simulink model "TP3_simulink"  (R2024a)
settings: Solver=VariableStepAuto  StartTime=0.0  StopTime=10  MaxStep=0.001  RelTol=1e-3
values from neighbouring files (symbols this model uses):
  A = [-1/(4*10^-3) -0.1/(4*10^-3) 0; 0.1/(2*10^-3) -(3*10^-3)/(2*10^-3) 0; 0 1 0]    [TP1.m]    (also in TP2.m = [0 1 0 0 0 0; -Kx/m -dx/m 0 0 0 0; 0 0 0 1 0 0; 0 0 -Ky/m -d; TP3.m = [0 1 0 0 0 0; -Kx/m -dx/m 0 0 0 0; 0 0 0 1 0 0; 0 0 -Ky/m -d)
  B = [1/(4*10^-3);0;0]    [TP1.m]    (also in TP2.m = [0 0 0; 1/m 0 0; 0 0 0; 0 1/m 0; 0 0 0; 0 0 1/m]; TP3.m = [0 0 0; 1/m 0 0; 0 0 0; 0 1/m 0; 0 0 0; 0 0 1/m])
  C = [0 0 1]    [TP1.m]    (also in TP2.m = [1 0 0 0 0 0; 0 0 1 0 0 0; 0 0 0 0 1 0]; TP3.m = [1 0 0 0 0 0; 0 0 1 0 0 0; 0 0 0 0 1 0])
  KxC = place(A(1:2,1:2),B(1:2,1),pcmdX)    [TP3.m]
  KyC = place(A(3:4,3:4),B(3:4,2),pcmdY)    [TP3.m]
  KzC = place(A(5:6,5:6),B(5:6,3),pcmdZ)    [TP3.m]
  L = [832330; 691770; 1550]    [TP1.m]    (also in TP2.m = (place(Aob.', C.', p)).'; TP3.m = (place(A.', C.', p)).')
settings Model: Creator=pedro.campos-afonso-  LastModifiedBy=pedro.campos-afonso-

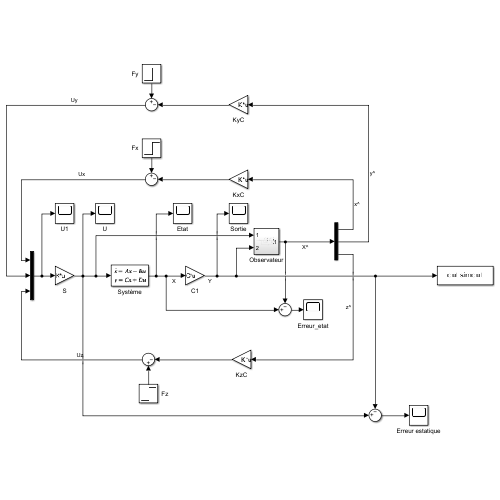
[thumbnail: Simulink's stored preview of the top-level diagram]
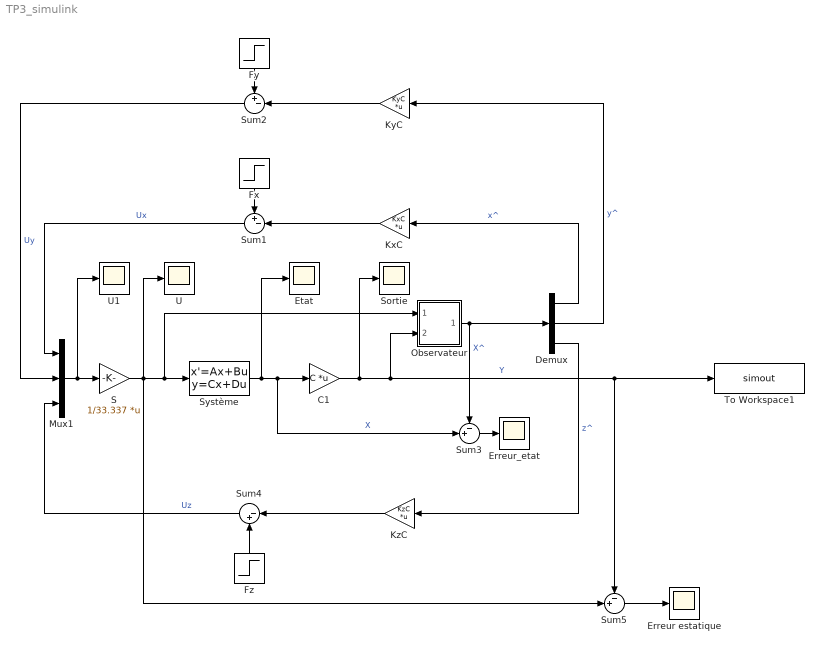
== system TP3_simulink ==
  C1 : Gain  Gain=C  Multiplication=Matrix(K*u)
  Demux : Demux  Outputs=3
  Erreur estatique : Scope
  Erreur_etat : Scope
  Etat : Scope
  Fx : Step  Time=0  SampleTime=0
  Fy : Step  Time=0  SampleTime=0
  Fz : Step  Time=0  SampleTime=0
  KxC : Gain  Gain=KxC  Multiplication=Matrix(K*u)
  KyC : Gain  Gain=KyC  Multiplication=Matrix(K*u)
  KzC : Gain  Gain=KzC  Multiplication=Matrix(K*u)
  Mux1 : Mux  Inputs=3
  Observateur : Subsystem
  S : Gain  Gain=1/33.337  Multiplication=Matrix(K*u)
  Sortie : Scope
  Sum1 : Sum  Inputs=+-|
  Sum2 : Sum  Inputs=+-|
  Sum3 : Sum  Inputs=-+|
  Sum4 : Sum  Inputs=|-+
  Sum5 : Sum  Inputs=-+|
  Système : StateSpace  A=A  B=B  C=eye(6)  D=zeros(6,3)  InitialCondition=[0.1; 0; 0.1; 0; -0.1; 0]
  To Workspace1 : ToWorkspace  VariableName=simout  SaveFormat=Timeseries  SampleTime=-1
  U : Scope
  U1 : Scope
  wires:
  C1/1 -> Sum5/1, To Workspace1/1, Observateur/2(In2), Sortie/1  "Y"
  Sum3/1 -> Erreur_etat/1
  Système/1 -> Sum3/2, C1/1, Etat/1  "X"
  Observateur/1(Out1) -> Demux/1, Sum3/1  "X^"
  Demux/1 -> KxC/1  "x^"
  Fx/1 -> Sum1/1
  KxC/1 -> Sum1/2
  Sum1/1 -> Mux1/1  "Ux"
  Demux/2 -> KyC/1  "y^"
  KyC/1 -> Sum2/2
  Fy/1 -> Sum2/1
  Sum2/1 -> Mux1/2  "Uy"
  Demux/3 -> KzC/1  "z^"
  Fz/1 -> Sum4/2
  KzC/1 -> Sum4/1
  Sum4/1 -> Mux1/3  "Uz"
  Sum5/1 -> Erreur estatique/1
  Mux1/1 -> S/1, U1/1
  S/1 -> Observateur/1(In1), Système/1, U/1, Sum5/2

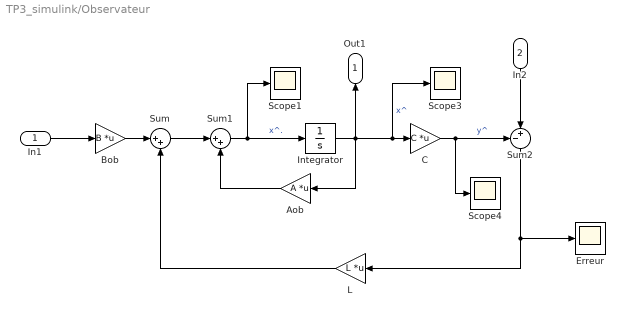
== system TP3_simulink/Observateur ==
  In1 : Inport
  In2 : Inport  Port=2
  Aob : Gain  Gain=A  Multiplication=Matrix(K*u)
  Bob : Gain  Gain=B  Multiplication=Matrix(K*u)
  C : Gain  Gain=C  Multiplication=Matrix(K*u)
  Erreur : Scope
  Integrator : Integrator
  L : Gain  Gain=L  Multiplication=Matrix(K*u)
  Scope1 : Scope
  Scope3 : Scope
  Scope4 : Scope
  Sum : Sum  Inputs=|++
  Sum1 : Sum  Inputs=|++
  Sum2 : Sum  Inputs=-+|
  Out1 : Outport
  wires:
  L/1 -> Sum/2
  Integrator/1 -> Out1/1, Aob/1, Scope3/1, C/1  "x^"
  Bob/1 -> Sum/1
  In2/1 -> Sum2/2
  Sum2/1 -> Erreur/1, L/1
  Sum/1 -> Sum1/1
  Aob/1 -> Sum1/2
  C/1 -> Sum2/1, Scope4/1  "y^"
  Sum1/1 -> Scope1/1, Integrator/1  "x^."
  In1/1 -> Bob/1
